simulink model "BuckBoostConverter"  (R2024a)
settings: Solver=VariableStepAuto  StartTime=0.0  StopTime=0.035  MaxStep=1e-4  RelTol=1e-4  EnableMultiTasking=on
libraries: spsSeriesRLCBranchLib x6, spsVoltageMeasurementLib x4, spsDiodeLib x3, spsCurrentMeasurementLib x2, spsMosfetLib x2, spsDCVoltageSourceLib x2, spsIGBTLib x1, spsPWMGeneratorDCDCLib x1, spspowerguiLib x1
settings Model: Creator=The MathWorks, Inc.  LastModifiedBy=ASUS
settings SolverCC: AlgebraicLoopSolver=TrustRegion  SolverResetMethod=Robust
settings DataIOCC: ReturnWorkspaceOutputs=off
settings OptimizationCC: EfficientFloat2IntCast=on  LifeSpan=inf
settings DebuggingCC: UnconnectedInputMsg=warning  UnconnectedOutputMsg=warning  UnconnectedLineMsg=warning  UniqueDataStoreMsg=error  StrictBusMsg=ErrorOnBusTreatedAsVector  SFUnexpectedBacktrackingDiag=warning  SFNoUnconditionalDefaultTransitionDiag=warning  SFExecutionAtInitializationDiag=none  ArithmeticOperatorsInVariantConditions=warning
settings ModelReferenceCC: EnableRefExpFcnMdlSchedulingChecks=on
settings SFSimCC: SimUseLocalCustomCode=off  CustomCodeUndefinedFunction=UseInterfaceOnly
settings RTWCC: RTWUseLocalCustomCode=off  GPUComputeCapability=3.5
settings CodeAppCC: StateflowObjectComments=on
settings GRTTargetCC: TargetLangStandard=C89/C90 (ANSI)
settings ConfigComp: CovMetricSettings=dw  CovSaveCumulativeToWorkspaceVar=on  CovSaveSingleToWorkspaceVar=on  CovExternalEMLEnable=off
settings SimscapeCC: SimscapeNormalizeSystem=off  SimscapeNominalValues={1, 'bar'; 1, 'cm^3/s'; 1, 'bar*kg/s'; 1, 'kJ/kg'; 1, 'kW'; }

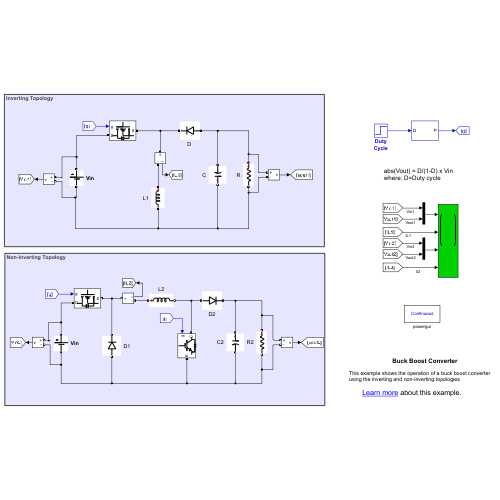
[thumbnail: Simulink's stored preview of the top-level diagram]
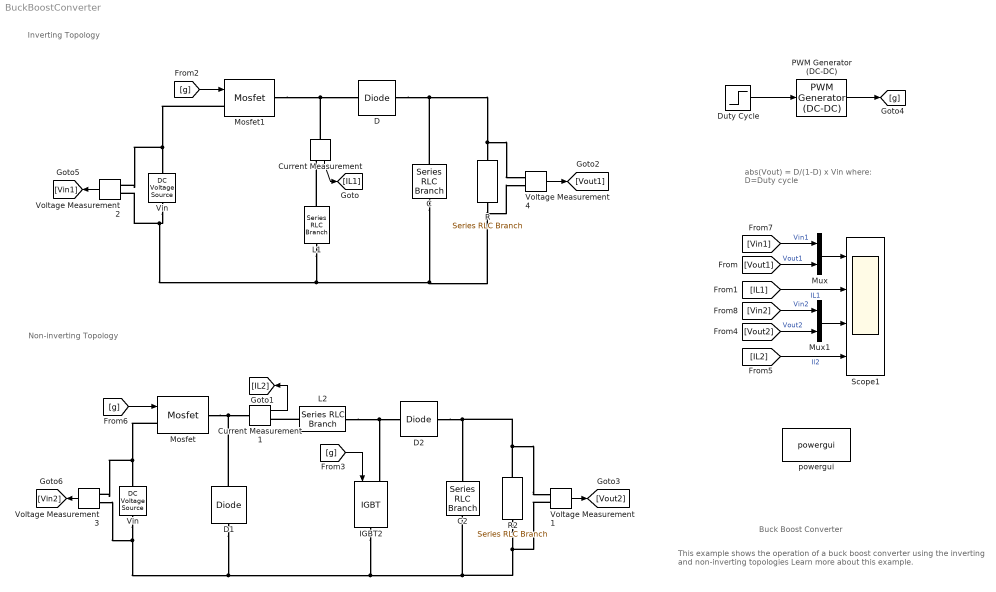
== system BuckBoostConverter ==
  note: abs(Vout) = D/(1-D) x Vin
      | where: D=Duty cycle
  note: Non-inverting Topology
  note: Inverting Topology
  note: This example shows the operation of a buck boost converter
      | using the inverting and non-inverting topologies
      |
      | Learn more about this example.
  note: Buck Boost Converter
  C : spsSeriesRLCBranchLib/Series RLC Branch  LConnTagsString=__new0  RConnTagsString=__new0  BranchType=C  Resistance=1e-4  Inductance=200e-6  SetiL0=off  InitialCurrent=0  Capacitance=2000e-6  Setx0=on  InitialVoltage=7.5  Measurements=None
  C2 : spsSeriesRLCBranchLib/Series RLC Branch  LConnTagsString=__new0  RConnTagsString=__new0  BranchType=C  Resistance=1e-4  Inductance=200e-6  SetiL0=off  InitialCurrent=0  Capacitance=2000e-6  Setx0=on  InitialVoltage=7.5  Measurements=None
  Current Measurement : spsCurrentMeasurementLib/Current Measurement  PhasorSimulation=off  OutputType=Complex  PSBequivalent=0
  Current Measurement1 : spsCurrentMeasurementLib/Current Measurement  PhasorSimulation=off  OutputType=Complex  PSBequivalent=0
  "D " : spsDiodeLib/Diode  Ron=1e-3  Lon=0  Vf=0  IC=0  UseSnubber=off  Rs=inf  Cs=inf  Measurements=off
  D1 : spsDiodeLib/Diode  Ron=1e-3  Lon=0  Vf=0  IC=0  UseSnubber=off  Rs=inf  Cs=inf  Measurements=off
  D2 : spsDiodeLib/Diode  Ron=1e-3  Lon=0  Vf=0  IC=0  UseSnubber=off  Rs=inf  Cs=inf  Measurements=off
  Duty Cycle : Step  Time=0.015  Before=0.456  After=0.528  SampleTime=0
  IGBT2 : spsIGBTLib/IGBT  Ron=0.001  Lon=0  Vf=0  Tf=1e-6  Tt=2e-6  IC=0  Rs=1e6  Cs=inf  Measurements=off
  L1 : spsSeriesRLCBranchLib/Series RLC Branch  LConnTagsString=__new0  RConnTagsString=__new0  BranchType=L  Resistance=1e-4  Inductance=750e-6  SetiL0=on  InitialCurrent=14  Capacitance=30e-6  Setx0=off  InitialVoltage=150  Measurements=None
  L2 : spsSeriesRLCBranchLib/Series RLC Branch  LConnTagsString=__new0  RConnTagsString=__new0  BranchType=L  Resistance=1e-4  Inductance=750e-6  SetiL0=on  InitialCurrent=14  Capacitance=30e-6  Setx0=off  InitialVoltage=150  Measurements=None
  Mosfet : spsMosfetLib/Mosfet  Ron=1e-3  Lon=0  Rd=1e-3  Vfd=0  IC=0  Rs=1e6  Cs=inf  Measurements=off
  Mosfet1 : spsMosfetLib/Mosfet  Ron=1e-3  Lon=0  Rd=1e-3  Vfd=0  IC=0  Rs=1e6  Cs=inf  Measurements=off
  Mux : Mux  Inputs=2
  Mux1 : Mux  Inputs=2
  PWM Generator (DC-DC) : spsPWMGeneratorDCDCLib/PWM Generator (DC-DC)  Fsw=10e3  Ts=0
  R : spsSeriesRLCBranchLib/Series RLC Branch  LConnTagsString=__new0  RConnTagsString=__new0  BranchType=R  Resistance=1  Inductance=200e-6  SetiL0=off  InitialCurrent=0  Capacitance=400e-6  Setx0=off  InitialVoltage=0  Measurements=None
  R2 : spsSeriesRLCBranchLib/Series RLC Branch  LConnTagsString=__new0  RConnTagsString=__new0  BranchType=R  Resistance=1  Inductance=200e-6  SetiL0=off  InitialCurrent=0  Capacitance=400e-6  Setx0=off  InitialVoltage=0  Measurements=None
  Scope1 : Scope  NumInputPorts=4
  Vin : spsDCVoltageSourceLib/DC Voltage Source  Amplitude=9  Measurements=None
  "Vin " : spsDCVoltageSourceLib/DC Voltage Source  Amplitude=9  Measurements=None
  Voltage Measurement{1..4} (4 alike) : spsVoltageMeasurementLib/Voltage Measurement  PhasorSimulation=off  OutputType=Complex  PSBequivalent=0
  powergui : spspowerguiLib/powergui  Priority=1  SimulationMode=Continuous  SampleTime=50e-6  frequency=60  Iterations=50  frequencyindice=0  Pbase=100e6  ErrMax=1e-4  UnitsV=kV  UnitsW=MW  buscounter=0  FunctionMessages=off  echomessages=off  EnableUseOfTLC=off  CurrentSourceSwitches=off  DisableSnubberDevices=off  DisableRonSwitches=off  DisableVfSwitches=off  DisplayEquations=off  AutomaticDiscreteSolvers=off  SolverType=Tustin/Backward Euler (TBE)  Interpol=off  ExternalGateDelay=off  methode=off  Ts=100  x0status=blocks  SPID=on  SwTol=0  HookPort=off  NonlinearTolerance=1e-4  nMaxIteration=100  ContinueOnMaxIteration=off  RestoreLinks=warning  ResistiveCurrentMeasurement=off  Frange=[0:2:500]  Ylog=off  Xlog=on  ShowGrid=off  save=off  variable=ZData  structure=0  ZoomFFT=off  StartTime=0.0  cycles=1  DisplayStyle=1  fundamental=60  FreqAxis=off  MaxFrequency=1000  frequencyindicesteady=1  RmsSteady=1  display=off
  wires:
  Current Measurement/1 -> [IL1]
  [IL1] -> Scope1/2  "IL1"
  [IL2] -> Scope1/4  "Il2"
  Duty Cycle/1 -> PWM Generator (DC-DC)/1
  Voltage Measurement1/1 -> [Vout2]
  [g] -> Mosfet/1
  Current Measurement1/1 -> [IL2]
  PWM Generator (DC-DC)/1 -> [g]
  [g] -> IGBT2/1
  [g] -> Mosfet1/1
  [Vout1] -> Mux/2  "Vout1"
  [Vin1] -> Mux/1  "Vin1"
  Mux/1 -> Scope1/1
  Voltage Measurement4/1 -> [Vout1]
  Voltage Measurement2/1 -> [Vin1]
  Mux1/1 -> Scope1/3
  [Vout2] -> Mux1/2  "Vout2"
  [Vin2] -> Mux1/1  "Vin2"
  Voltage Measurement3/1 -> [Vin2]
  connections:
  "Vin "/LConn1 -- R/RConn1 -- Voltage Measurement4/LConn2 -- C/LConn1 -- L1/RConn1 -- Voltage Measurement2/LConn2
  "D "/LConn1 -- C/RConn1 -- Voltage Measurement4/LConn1 -- R/LConn1
  Mosfet1/LConn1 -- Voltage Measurement2/LConn1 -- "Vin "/RConn1
  Current Measurement/LConn1 -- Mosfet1/RConn1 -- "D "/RConn1
  L1/LConn1 -- Current Measurement/RConn1
  Vin/LConn1 -- Voltage Measurement3/LConn2 -- D1/LConn1 -- Voltage Measurement1/LConn2 -- R2/RConn1 -- C2/RConn1 -- IGBT2/RConn1
  D2/RConn1 -- Voltage Measurement1/LConn1 -- R2/LConn1 -- C2/LConn1
  Mosfet/LConn1 -- Voltage Measurement3/LConn1 -- Vin/RConn1
  L2/RConn1 -- IGBT2/LConn1 -- D2/LConn1
  L2/LConn1 -- Current Measurement1/RConn1
  Mosfet/RConn1 -- D1/RConn1 -- Current Measurement1/LConn1
